simulink model "Filter_plus_damper_R2016a"  (R2016a)
settings: Solver=FixedStepDiscrete  SolverMode=SingleTasking  StartTime=0.0  StopTime=0.6  FixedStep=Ts  RelTol=1e-3
InitFcn:
  | Ts=5e-6;
  | f=60;
  | w=2*pi*f;
libraries: powerlib x25, powerlib_meascontrol x4
settings Model: Creator=Aminsystem  LastModifiedBy=Aminsystem
settings DataIOCC: SaveOutput=off  SignalLogging=off  DSMLogging=off  SaveTime=off
settings DebuggingCC: UnconnectedInputMsg=none  UnconnectedOutputMsg=none  UnconnectedLineMsg=none  SFUnexpectedBacktrackingDiag=error  SFNoUnconditionalDefaultTransitionDiag=error
settings ModelReferenceCC: EnableRefExpFcnMdlSchedulingChecks=off
settings SFSimCC: SimUseLocalCustomCode=on
settings RTWCC: Description=Generic Real-Time Target  RTWUseLocalCustomCode=on
settings GRTTargetCC: TargetLangStandard=C99 (ISO)
settings ConfigComp: CovMetricSettings=dwe  CovSaveCumulativeToWorkspaceVar=off  CovSaveSingleToWorkspaceVar=off  CovExternalEMLEnable=on

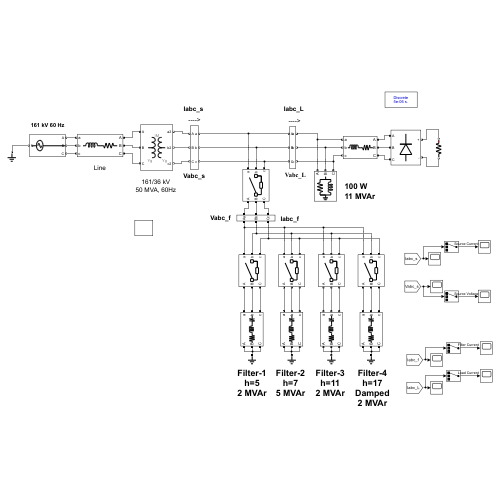
[thumbnail: Simulink's stored preview of the top-level diagram]
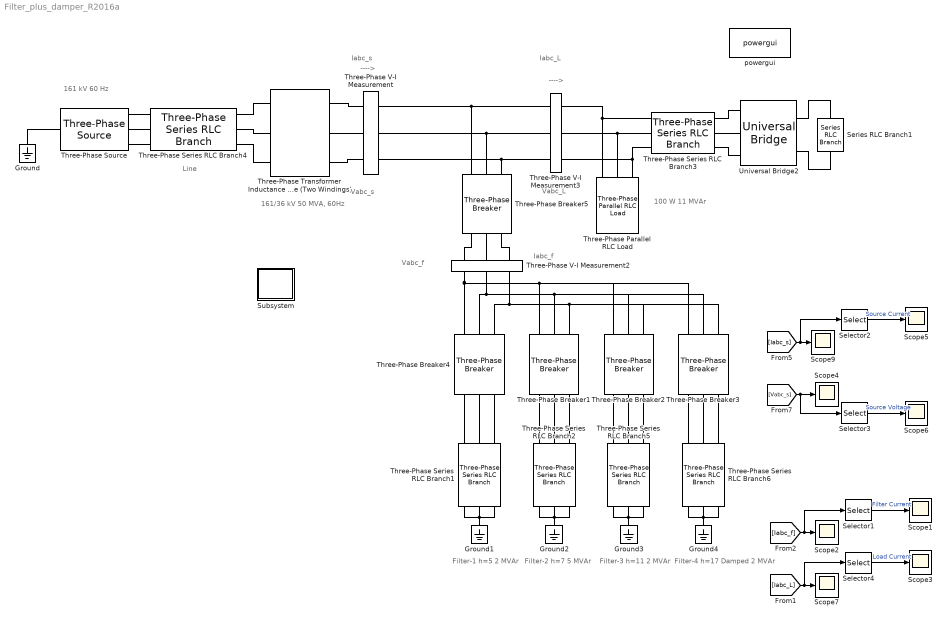
== system Filter_plus_damper_R2016a ==
  note: Line
  note: Filter-1
      | h=5
      | 2 MVAr
  note: 100 W
      | 11 MVAr
  note: 161 kV 60 Hz
  note: Iabc_L
  note: Vabc_s
  note: Iabc_s
  note: ---->
  note: ---->
  note: Vabc_L
  note: Iabc_f
  note: Vabc_f
  note: 161/36 kV
      | 50 MVA, 60Hz
  note: Filter-2
      | h=7
      | 5 MVAr
  note: Filter-3
      | h=11
      | 2 MVAr
  note: Filter-4
      | h=17
      | Damped
      | 2 MVAr
  Ground{,1..4} (5 alike) : powerlib/Elements/Ground  LConnTagsString=a
  Scope{1..7,9} (8 alike) : Scope
  Selector{1..4} (4 alike) : Selector  InputPortWidth=3  IndexOptions=Index vector (dialog)  Indices=[1]  OutputSizes=1
  Series RLC Branch1 : powerlib/Elements/Series RLC Branch  LConnTagsString=__new0  RConnTagsString=__new0  BranchType=R  Resistance=36e3*36e3/20e6  Inductance=0.5e-3  SetiL0=off  InitialCurrent=0  Capacitance=1e-6  Setx0=off  InitialVoltage=0  Measurements=None
  Subsystem : Subsystem
  Three-Phase Parallel RLC Load : powerlib/Elements/Three-Phase Parallel RLC Load  LConnTagsString=A|B|C  Configuration=Y (grounded)  NominalVoltage=36e3  Vabc=[1e3 1e3 1e3]  Vabcp=[1e3 1e3 1e3]  NominalFrequency=50  UnbalancedPower=off  ActivePower=100  InductivePower=11e6  CapacitivePower=0  Pabc=[10e3 9e3 11e3]  QLabc=[100 90 110]  QCabc=[100 90 110]  Pabcp=[10e3 9e3 11e3]  QLabcp=[100 90 110]  QCabcp=[100 90 110]  Measurements=None  LoadType=constant Z
  Three-Phase Series RLC Branch1 : powerlib/Elements/Three-Phase Series RLC Branch  LConnTagsString=A|B|C  RConnTagsString=A|B|C  BranchType=RLC  Resistance=36e3*36e3/2e6/5/100  Inductance=36e3*36e3/2e6/5/5/w  Capacitance=2e6/(36e3*36e3*w)  Measurements=None
  Three-Phase Series RLC Branch2 : powerlib/Elements/Three-Phase Series RLC Branch  LConnTagsString=A|B|C  RConnTagsString=A|B|C  BranchType=RLC  Resistance=36e3*36e3/5e6/7/100  Inductance=36e3*36e3/5e6/7/7/w  Capacitance=5e6/(36e3*36e3*w)  Measurements=None
  Three-Phase Series RLC Branch3 : powerlib/Elements/Three-Phase Series RLC Branch  LConnTagsString=A|B|C  RConnTagsString=A|B|C  BranchType=RL  Resistance=0.1e-3/(90*90)  Inductance=0.1e-3/(90*90)  Capacitance=1e-6  Measurements=None
  Three-Phase Series RLC Branch4 : powerlib/Elements/Three-Phase Series RLC Branch  LConnTagsString=A|B|C  RConnTagsString=A|B|C  BranchType=RL  Resistance=1/(8*8)  Inductance=16e-3/(8*8)  Capacitance=1e-6  Measurements=None
  Three-Phase Series RLC Branch5 : powerlib/Elements/Three-Phase Series RLC Branch  LConnTagsString=A|B|C  RConnTagsString=A|B|C  BranchType=RLC  Resistance=36e3*36e3/2e6/11/100  Inductance=36e3*36e3/2e6/11/11/w  Capacitance=2e6/(36e3*36e3*w)  Measurements=None
  Three-Phase Series RLC Branch6 : powerlib/Elements/Three-Phase Series RLC Branch  LConnTagsString=A|B|C  RConnTagsString=A|B|C  BranchType=RLC  Resistance=36e3*36e3/5e6/17/5  Inductance=36e3*36e3/5e6/17/17/w  Capacitance=5e6/(36e3*36e3*w)  Measurements=None
  Three-Phase V-I Measurement : powerlib/Measurements/Three-Phase V-I Measurement  VoltageMeasurement=phase-to-ground  SetLabelV=on  LabelV=Vabc_s  Vpu=off  VpuLL=off  CurrentMeasurement=yes  SetLabelI=on  LabelI=Iabc_s  Ipu=off  Pbase=100e6  Vbase=500e3  OutputType=Complex  PhasorSimulation=off  PSBequivalent=0
  Three-Phase V-I Measurement2 : powerlib/Measurements/Three-Phase V-I Measurement  VoltageMeasurement=phase-to-ground  SetLabelV=on  LabelV=Vabc_f  Vpu=off  VpuLL=off  CurrentMeasurement=yes  SetLabelI=on  LabelI=Iabc_f  Ipu=off  Pbase=100e6  Vbase=500e3  OutputType=Complex  PhasorSimulation=off  PSBequivalent=0
  Three-Phase V-I Measurement3 : powerlib/Measurements/Three-Phase V-I Measurement  VoltageMeasurement=phase-to-ground  SetLabelV=on  LabelV=Vabc_L  Vpu=off  VpuLL=off  CurrentMeasurement=yes  SetLabelI=on  LabelI=Iabc_L  Ipu=off  Pbase=100e6  Vbase=500e3  OutputType=Complex  PhasorSimulation=off  PSBequivalent=0
  Three-Phase Breaker1 : powerlib/Elements/Three-Phase Breaker  InitialState=open  SwitchA=on  SwitchB=on  SwitchC=on  SwitchTimes=[0.25]  External=off  BreakerResistance=0.001  SnubberResistance=1e7  SnubberCapacitance=inf  Measurements=None
  Three-Phase Breaker2 : powerlib/Elements/Three-Phase Breaker  InitialState=open  SwitchA=on  SwitchB=on  SwitchC=on  SwitchTimes=[0.3]  External=off  BreakerResistance=0.001  SnubberResistance=1e7  SnubberCapacitance=inf  Measurements=None
  Three-Phase Breaker3 : powerlib/Elements/Three-Phase Breaker  InitialState=open  SwitchA=on  SwitchB=on  SwitchC=on  SwitchTimes=[0.35]  External=off  BreakerResistance=0.001  SnubberResistance=1e7  SnubberCapacitance=inf  Measurements=None
  Three-Phase Breaker4 : powerlib/Elements/Three-Phase Breaker  InitialState=open  SwitchA=on  SwitchB=on  SwitchC=on  SwitchTimes=[0.2]  External=off  BreakerResistance=0.001  SnubberResistance=1e7  SnubberCapacitance=inf  Measurements=None
  Three-Phase Breaker5 : powerlib/Elements/Three-Phase Breaker  InitialState=open  SwitchA=on  SwitchB=on  SwitchC=on  SwitchTimes=[0.2]  External=off  BreakerResistance=0.001  SnubberResistance=1e7  SnubberCapacitance=inf  Measurements=None
  Three-Phase Source : powerlib/Electrical Sources/Three-Phase Source  InternalConnection=Yn  VoltagePhases=off  Voltage=161e3  PhaseAngle=0  Voltage_phases=[25e3 25e3 25e3]/sqrt(3)  PhaseAngles_phases=[0 -120 +120]  Frequency=f  NonIdealSource=off  SpecifyImpedance=off  Resistance=0.8929  Inductance=16.58e-3  ShortCircuitLevel=100e6  BaseVoltage=20e3  XRratio=10  BusType=swing  Pref=10e3  Qref=0  Prefabc=[10e3, 10e3, 10e3]  Qrefabc=[0, 0, 0]  Qmin=-inf  Qmax=inf
  Three-Phase Transformer Inductance Matrix Type (Two Windings) : powerlib/Elements/Three-Phase Transformer Inductance Matrix Type (Two Windings)  CoreType=Three single-phase cores  Winding1Connection=Yg  Winding2Connection=Yg  AutoTransformer=off  Measurements=None  NominalPower=[50e6, f]  VLLnom=[161e3, 36e3]  WindingResistances=[0.01, 0.01]  NoLoadIexcPos=2  NoLoadPlossPos=250  ShortCircuitReactancePos=0.06  ShortCircuitReactancePosAuto=0.06  NoLoadIexcZero=100  NoLoadPlossZero=1500  ShortCircuitReactanceZero=0.03  ShortCircuitReactanceZeroAuto=0.03
  Universal Bridge2 : powerlib/Power Electronics/Universal Bridge  Arms=3  SnubberResistance=1e5  SnubberCapacitance=inf  Device=Diodes  Ron=1e-3  Lon=0  ForwardVoltages="[  0  0  ]"  ForwardVoltage=0  GTOparameters=[ 10e-6 , 20e-6 ]  IGBTparameters=[ 1e-6 , 2e-6 ]  Measurements=None  Measurements_2=None  converterType=Rectifier
  powergui : powerlib/powergui  Priority=1  SimulationMode=Discrete  SampleTime=Ts  frequency=60  Iterations=50  frequencyindice=0  Pbase=100e6  ErrMax=1e-4  UnitsV=kV  UnitsW=MW  buscounter=0  FunctionMessages=off  echomessages=off  EnableUseOfTLC=off  CurrentSourceSwitches=off  DisableSnubberDevices=off  DisableRonSwitches=off  DisableVfSwitches=off  DisplayEquations=off  AutomaticDiscreteSolvers=off  SolverType=Tustin  Interpol=off  ExternalGateDelay=off  methode=off  Ts=100  x0status=blocks  SPID=on  SwTol=0  HookPort=off  NonlinearTolerance=1e-4  nMaxIteration=100  ContinueOnMaxIteration=off  RestoreLinks=warning  ResistiveCurrentMeasurement=off  Frange=[0:2:500]  Ylog=off  Xlog=on  ShowGrid=off  save=off  variable=ZData  structure=Iabc_s  ZoomFFT=off  StartTime=1.6  cycles=20  DisplayStyle=1  fundamental=50  FreqAxis=on  MaxFrequency=50*20  frequencyindicesteady=1  RmsSteady=1  display=off
  wires:
  [Iabc_s] -> Selector2/1, Scope9/1
  Selector2/1 -> Scope5/1  "Source Current"
  [Vabc_s] -> Scope4/1, Selector3/1
  Selector3/1 -> Scope6/1  "Source Voltage"
  Selector1/1 -> Scope1/1  "Filter Current"
  [Iabc_f] -> Scope2/1, Selector1/1
  [Iabc_L] -> Selector4/1, Scope7/1
  Selector4/1 -> Scope3/1  "Load Current"
  connections:
  Three-Phase Series RLC Branch3/RConn2 -- Three-Phase Parallel RLC Load/LConn2 -- Three-Phase V-I Measurement3/RConn2
  Three-Phase Breaker5/LConn1 -- Three-Phase V-I Measurement2/RConn1
  Three-Phase V-I Measurement3/RConn3 -- Three-Phase Parallel RLC Load/LConn3 -- Three-Phase Series RLC Branch3/RConn3
  Three-Phase Series RLC Branch3/RConn1 -- Three-Phase Parallel RLC Load/LConn1 -- Three-Phase V-I Measurement3/RConn1
  Three-Phase Breaker5/LConn2 -- Three-Phase V-I Measurement2/RConn2
  Three-Phase V-I Measurement/RConn3 -- Three-Phase Breaker5/RConn3 -- Three-Phase V-I Measurement3/LConn3
  Ground/LConn1 -- Three-Phase Source/LConn1
  Three-Phase Breaker5/LConn3 -- Three-Phase V-I Measurement2/RConn3
  Three-Phase V-I Measurement/RConn1 -- Three-Phase Breaker5/RConn1 -- Three-Phase V-I Measurement3/LConn1
  Three-Phase V-I Measurement/RConn2 -- Three-Phase Breaker5/RConn2 -- Three-Phase V-I Measurement3/LConn2
  Three-Phase Breaker2/RConn2 -- Three-Phase Breaker3/RConn2 -- Three-Phase Breaker1/RConn2 -- Three-Phase Breaker4/RConn2 -- Three-Phase V-I Measurement2/LConn2
  Three-Phase V-I Measurement2/LConn1 -- Three-Phase Breaker4/RConn1 -- Three-Phase Breaker3/RConn1 -- Three-Phase Breaker2/RConn1 -- Three-Phase Breaker1/RConn1
  Three-Phase Breaker3/RConn3 -- Three-Phase Breaker2/RConn3 -- Three-Phase Breaker1/RConn3 -- Three-Phase Breaker4/RConn3 -- Three-Phase V-I Measurement2/LConn3
  Three-Phase Series RLC Branch4/RConn1 -- Three-Phase Source/RConn1
  Three-Phase Series RLC Branch4/RConn3 -- Three-Phase Source/RConn3
  Three-Phase Series RLC Branch4/RConn2 -- Three-Phase Source/RConn2
  Three-Phase Transformer Inductance Matrix Type (Two Windings)/LConn2 -- Three-Phase Series RLC Branch4/LConn2
  Three-Phase Transformer Inductance Matrix Type (Two Windings)/LConn1 -- Three-Phase Series RLC Branch4/LConn1
  Three-Phase Transformer Inductance Matrix Type (Two Windings)/LConn3 -- Three-Phase Series RLC Branch4/LConn3
  Three-Phase Transformer Inductance Matrix Type (Two Windings)/RConn1 -- Three-Phase V-I Measurement/LConn1
  Three-Phase Transformer Inductance Matrix Type (Two Windings)/RConn2 -- Three-Phase V-I Measurement/LConn2
  Three-Phase Transformer Inductance Matrix Type (Two Windings)/RConn3 -- Three-Phase V-I Measurement/LConn3
  Ground2/LConn1 -- Three-Phase Series RLC Branch2/LConn1 -- Three-Phase Series RLC Branch2/LConn3 -- Three-Phase Series RLC Branch2/LConn2
  Three-Phase Series RLC Branch2/RConn1 -- Three-Phase Breaker1/LConn1
  Three-Phase Series RLC Branch2/RConn2 -- Three-Phase Breaker1/LConn2
  Three-Phase Series RLC Branch2/RConn3 -- Three-Phase Breaker1/LConn3
  Three-Phase Series RLC Branch5/RConn1 -- Three-Phase Breaker2/LConn1
  Three-Phase Series RLC Branch5/RConn2 -- Three-Phase Breaker2/LConn2
  Three-Phase Series RLC Branch5/RConn3 -- Three-Phase Breaker2/LConn3
  Three-Phase Series RLC Branch6/RConn1 -- Three-Phase Breaker3/LConn1
  Three-Phase Series RLC Branch6/RConn2 -- Three-Phase Breaker3/LConn2
  Three-Phase Series RLC Branch6/RConn3 -- Three-Phase Breaker3/LConn3
  Three-Phase Series RLC Branch1/RConn1 -- Three-Phase Breaker4/LConn1
  Three-Phase Series RLC Branch1/RConn2 -- Three-Phase Breaker4/LConn2
  Three-Phase Series RLC Branch1/RConn3 -- Three-Phase Breaker4/LConn3
  Universal Bridge2/RConn1 -- Series RLC Branch1/LConn1
  Series RLC Branch1/RConn1 -- Universal Bridge2/RConn2
  Three-Phase Series RLC Branch3/LConn2 -- Universal Bridge2/LConn2
  Three-Phase Series RLC Branch3/LConn1 -- Universal Bridge2/LConn1
  Three-Phase Series RLC Branch3/LConn3 -- Universal Bridge2/LConn3
  Three-Phase Series RLC Branch5/LConn2 -- Ground3/LConn1 -- Three-Phase Series RLC Branch5/LConn1 -- Three-Phase Series RLC Branch5/LConn3
  Three-Phase Series RLC Branch6/LConn2 -- Ground4/LConn1 -- Three-Phase Series RLC Branch6/LConn1 -- Three-Phase Series RLC Branch6/LConn3
  Three-Phase Series RLC Branch1/LConn2 -- Ground1/LConn1 -- Three-Phase Series RLC Branch1/LConn1 -- Three-Phase Series RLC Branch1/LConn3

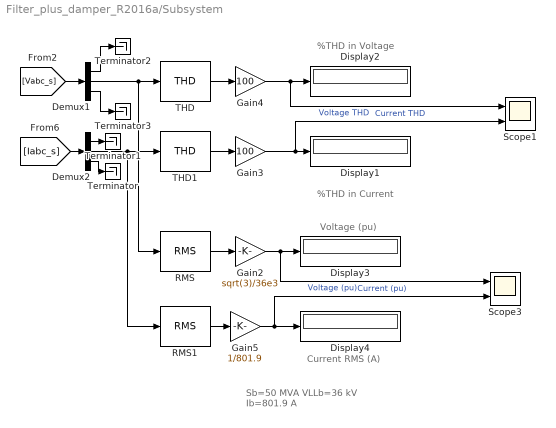
== system Filter_plus_damper_R2016a/Subsystem ==
  note: Sb=50 MVA
      | VLLb=36 kV
      | Ib=801.9 A
  note: %THD in Current
  note: %THD in Voltage
  note: Voltage (pu)
  note: Current RMS (A)
  Demux1 : Demux  Outputs=3
  Demux2 : Demux  Outputs=3
  Display{1..4} (4 alike) : Display
  Gain2 : Gain  Gain=sqrt(3)/36e3
  Gain3 : Gain  Gain=100
  Gain4 : Gain  Gain=100
  Gain5 : Gain  Gain=1/801.9
  RMS : powerlib_meascontrol/Measurements/RMS  TrueRMS=on  Freq=f  RMSInit=0  Ts=Ts
  RMS1 : powerlib_meascontrol/Measurements/RMS  TrueRMS=on  Freq=f  RMSInit=0  Ts=Ts
  Scope1 : Scope  NumInputPorts=2
  Scope3 : Scope  NumInputPorts=2
  THD : powerlib_meascontrol/Measurements/THD  Freq=f  Ts=Ts
  THD1 : powerlib_meascontrol/Measurements/THD  Freq=f  Ts=Ts
  Terminator{,1..3} (4 alike) : Terminator
  wires:
  Demux1/2 -> RMS/1, THD/1
  [Iabc_s] -> Demux2/1
  THD/1 -> Gain4/1
  Gain3/1 -> Scope1/2, Display1/1  "Current THD"
  THD1/1 -> Gain3/1
  Demux2/2 -> RMS1/1, THD1/1
  [Vabc_s] -> Demux1/1
  Gain5/1 -> Scope3/2, Display4/1  "Current (pu)"
  Gain4/1 -> Scope1/1, Display2/1  "Voltage THD"
  RMS/1 -> Gain2/1
  RMS1/1 -> Gain5/1
  Gain2/1 -> Scope3/1, Display3/1  "Voltage (pu)"
  Demux2/3 -> Terminator/1
  Demux2/1 -> Terminator1/1
  Demux1/1 -> Terminator2/1
  Demux1/3 -> Terminator3/1
